simulink model "pedalboys_finalfxchain"  (R2025b)
settings: Solver=VariableStepAuto  StartTime=0.0  StopTime=inf  FixedStep=44100  RelTol=1e-3
libraries: audiodynamicrange x2, audiosources x1, dspsnks4 x1
(part 2 of 2)

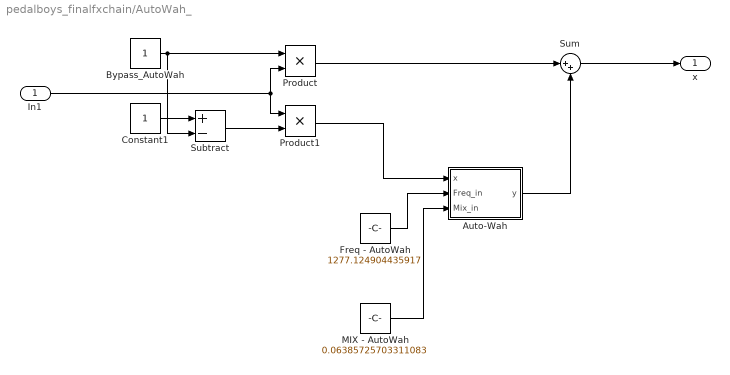
== system pedalboys_finalfxchain/AutoWah_ ==
  In1 : Inport
  Auto-Wah : MATLAB Function  TreatAsAtomicUnit=on
  Bypass_AutoWah : Constant
  Constant1 : Constant
  Freq - AutoWah : Constant  Value=1277.124904435917
  MIX - AutoWah : Constant  Value=0.06385725703311083
  Product : Product
  Product1 : Product
  Subtract : Sum  Inputs=+-
  Sum : Sum  Inputs=|++
  x : Outport
  wires:
  Subtract/1 -> Product1/2
  Bypass_AutoWah/1 -> Product/1, Subtract/2
  Sum/1 -> x/1
  Auto-Wah/1(y) -> Sum/2
  Product/1 -> Sum/1
  In1/1 -> Product/2, Product1/1
  Constant1/1 -> Subtract/1
  Product1/1 -> Auto-Wah/1(x)
  MIX - AutoWah/1 -> Auto-Wah/3(Mix_in)
  Freq - AutoWah/1 -> Auto-Wah/2(Freq_in)

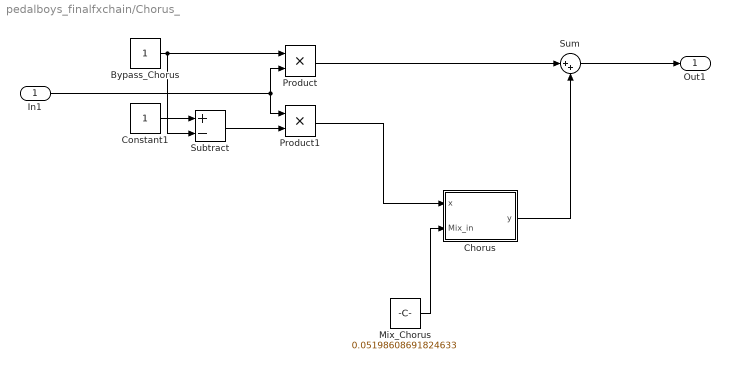
== system pedalboys_finalfxchain/Chorus_ ==
  In1 : Inport
  Bypass_Chorus : Constant
  Chorus : MATLAB Function  TreatAsAtomicUnit=on
  Constant1 : Constant
  Mix_Chorus : Constant  Value=0.05198608691824633
  Product : Product
  Product1 : Product
  Subtract : Sum  Inputs=+-
  Sum : Sum  Inputs=|++
  Out1 : Outport
  wires:
  Product1/1 -> Chorus/1(x)
  Subtract/1 -> Product1/2
  Bypass_Chorus/1 -> Product/1, Subtract/2
  Sum/1 -> Out1/1
  Chorus/1(y) -> Sum/2
  Product/1 -> Sum/1
  In1/1 -> Product/2, Product1/1
  Constant1/1 -> Subtract/1
  Mix_Chorus/1 -> Chorus/2(Mix_in)

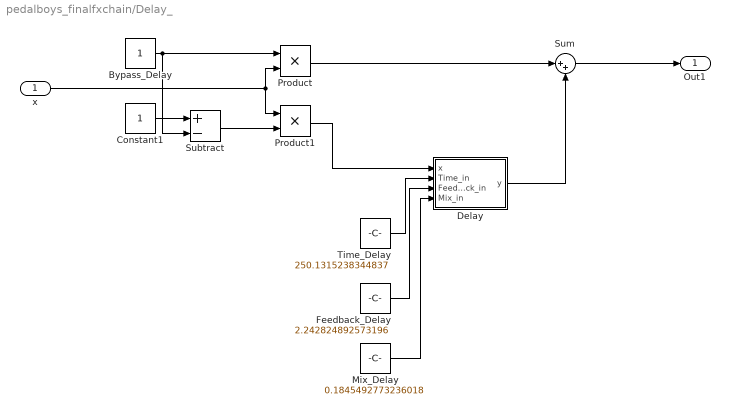
== system pedalboys_finalfxchain/Delay_ ==
  x : Inport
  Bypass_Delay : Constant
  Constant1 : Constant
  Delay : MATLAB Function  TreatAsAtomicUnit=on
  Feedback_Delay : Constant  Value=2.242824892573196
  Mix_Delay : Constant  Value=0.1845492773236018
  Product : Product
  Product1 : Product
  Subtract : Sum  Inputs=+-
  Sum : Sum  Inputs=|++
  Time_Delay : Constant  Value=250.1315238344837
  Out1 : Outport
  wires:
  Sum/1 -> Out1/1
  Product1/1 -> Delay/1(x)
  Product/1 -> Sum/1
  Bypass_Delay/1 -> Product/1, Subtract/2
  Constant1/1 -> Subtract/1
  x/1 -> Product/2, Product1/1
  Subtract/1 -> Product1/2
  Mix_Delay/1 -> Delay/4(Mix_in)
  Time_Delay/1 -> Delay/2(Time_in)
  Feedback_Delay/1 -> Delay/3(Feedback_in)
  Delay/1(y) -> Sum/2

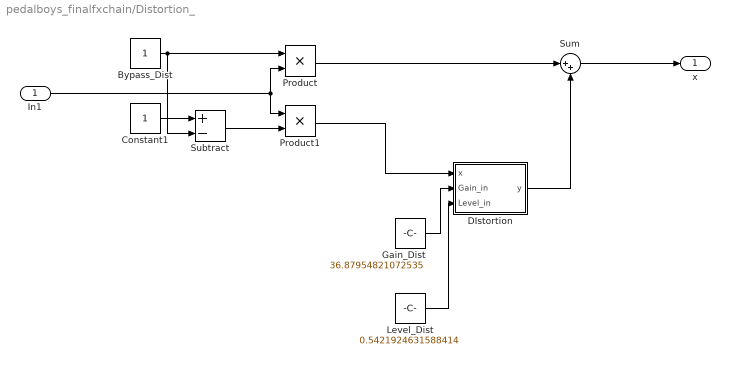
== system pedalboys_finalfxchain/Distortion_ ==
  In1 : Inport
  Bypass_Dist : Constant
  Constant1 : Constant
  DIstortion : MATLAB Function  TreatAsAtomicUnit=on
  Gain_Dist : Constant  Value=36.87954821072535
  Level_Dist : Constant  Value=0.5421924631588414
  Product : Product
  Product1 : Product
  Subtract : Sum  Inputs=+-
  Sum : Sum  Inputs=|++
  x : Outport
  wires:
  Product1/1 -> DIstortion/1(x)
  Subtract/1 -> Product1/2
  Bypass_Dist/1 -> Product/1, Subtract/2
  Sum/1 -> x/1
  DIstortion/1(y) -> Sum/2
  Product/1 -> Sum/1
  In1/1 -> Product/2, Product1/1
  Constant1/1 -> Subtract/1
  Gain_Dist/1 -> DIstortion/2(Gain_in)
  Level_Dist/1 -> DIstortion/3(Level_in)

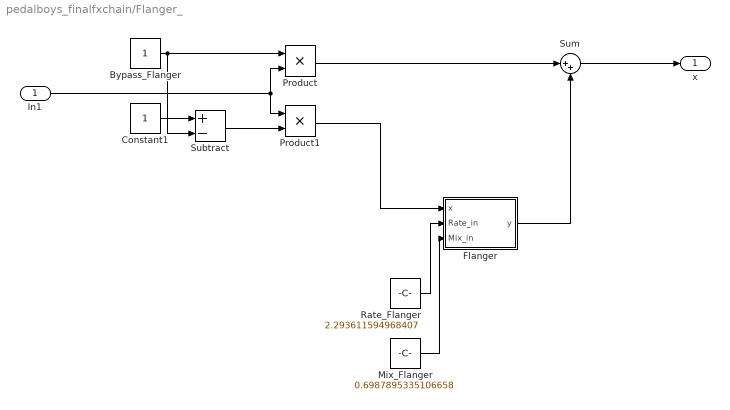
== system pedalboys_finalfxchain/Flanger_ ==
  In1 : Inport
  Bypass_Flanger : Constant
  Constant1 : Constant
  Flanger : MATLAB Function  TreatAsAtomicUnit=on
  Mix_Flanger : Constant  Value=0.6987895335106658
  Product : Product
  Product1 : Product
  Rate_Flanger : Constant  Value=2.293611594968407
  Subtract : Sum  Inputs=+-
  Sum : Sum  Inputs=|++
  x : Outport
  wires:
  Subtract/1 -> Product1/2
  Bypass_Flanger/1 -> Product/1, Subtract/2
  Sum/1 -> x/1
  Flanger/1(y) -> Sum/2
  Product/1 -> Sum/1
  In1/1 -> Product/2, Product1/1
  Constant1/1 -> Subtract/1
  Rate_Flanger/1 -> Flanger/2(Rate_in)
  Product1/1 -> Flanger/1(x)
  Mix_Flanger/1 -> Flanger/3(Mix_in)

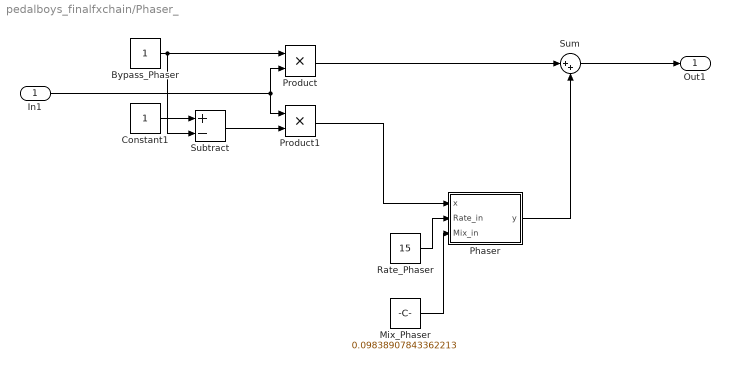
== system pedalboys_finalfxchain/Phaser_ ==
  In1 : Inport
  Bypass_Phaser : Constant
  Constant1 : Constant
  Mix_Phaser : Constant  Value=0.09838907843362213
  Phaser : MATLAB Function  TreatAsAtomicUnit=on
  Product : Product
  Product1 : Product
  Rate_Phaser : Constant  Value=15
  Subtract : Sum  Inputs=+-
  Sum : Sum  Inputs=|++
  Out1 : Outport
  wires:
  Product1/1 -> Phaser/1(x)
  Subtract/1 -> Product1/2
  Bypass_Phaser/1 -> Product/1, Subtract/2
  Sum/1 -> Out1/1
  Phaser/1(y) -> Sum/2
  Product/1 -> Sum/1
  In1/1 -> Product/2, Product1/1
  Constant1/1 -> Subtract/1
  Rate_Phaser/1 -> Phaser/2(Rate_in)
  Mix_Phaser/1 -> Phaser/3(Mix_in)

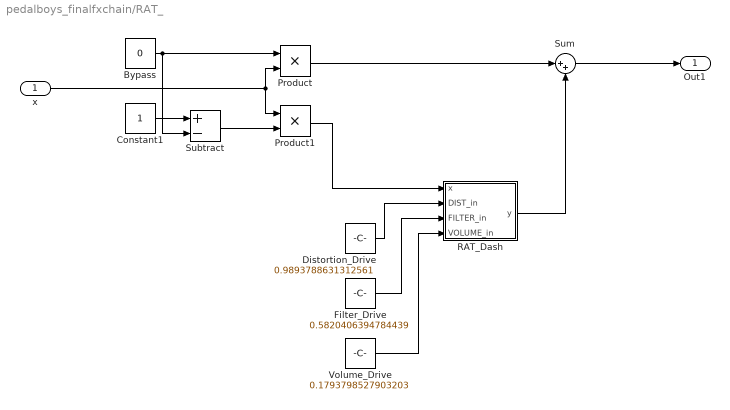
== system pedalboys_finalfxchain/RAT_ ==
  x : Inport
  Bypass : Constant  Value=0
  Constant1 : Constant
  Distortion_Drive : Constant  Value=0.9893788631312561
  Filter_Drive : Constant  Value=0.5820406394784439
  Product : Product
  Product1 : Product
  RAT_Dash : MATLAB Function  TreatAsAtomicUnit=on
  Subtract : Sum  Inputs=+-
  Sum : Sum  Inputs=|++
  Volume_Drive : Constant  Value=0.1793798527903203
  Out1 : Outport
  wires:
  Sum/1 -> Out1/1
  RAT_Dash/1(y) -> Sum/2
  Distortion_Drive/1 -> RAT_Dash/2(DIST_in)
  Volume_Drive/1 -> RAT_Dash/4(VOLUME_in)
  Filter_Drive/1 -> RAT_Dash/3(FILTER_in)
  Product1/1 -> RAT_Dash/1(x)
  Product/1 -> Sum/1
  Bypass/1 -> Product/1, Subtract/2
  Constant1/1 -> Subtract/1
  x/1 -> Product/2, Product1/1
  Subtract/1 -> Product1/2

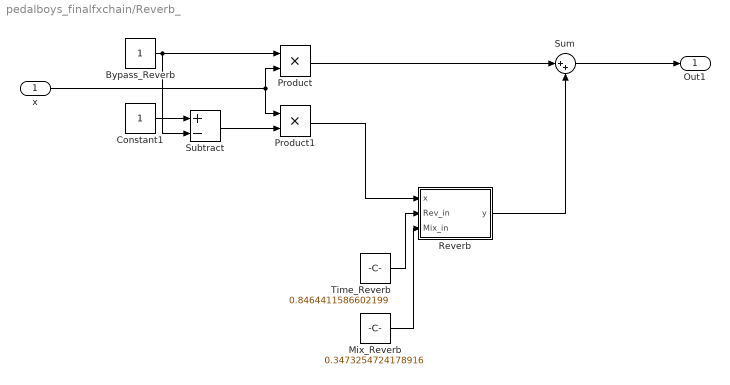
== system pedalboys_finalfxchain/Reverb_ ==
  x : Inport
  Bypass_Reverb : Constant
  Constant1 : Constant
  Mix_Reverb : Constant  Value=0.3473254724178916
  Product : Product
  Product1 : Product
  Reverb : MATLAB Function  TreatAsAtomicUnit=on
  Subtract : Sum  Inputs=+-
  Sum : Sum  Inputs=|++
  Time_Reverb : Constant  Value=0.8464411586602199
  Out1 : Outport
  wires:
  Sum/1 -> Out1/1
  Reverb/1(y) -> Sum/2
  Product1/1 -> Reverb/1(x)
  Product/1 -> Sum/1
  Bypass_Reverb/1 -> Product/1, Subtract/2
  Constant1/1 -> Subtract/1
  x/1 -> Product/2, Product1/1
  Subtract/1 -> Product1/2
  Time_Reverb/1 -> Reverb/2(Rev_in)
  Mix_Reverb/1 -> Reverb/3(Mix_in)

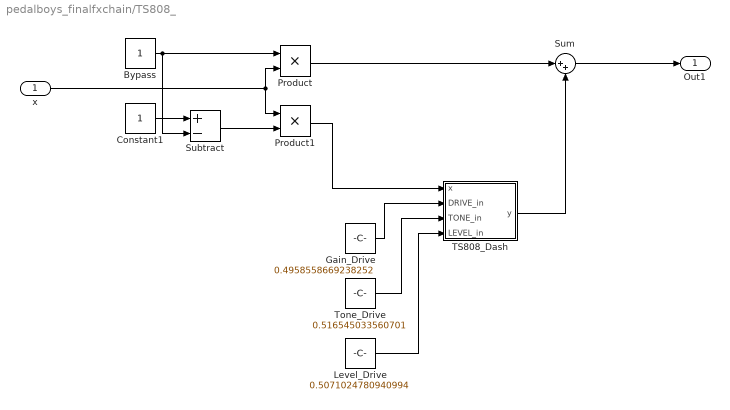
== system pedalboys_finalfxchain/TS808_ ==
  x : Inport
  Bypass : Constant
  Constant1 : Constant
  Gain_Drive : Constant  Value=0.4958558669238252
  Level_Drive : Constant  Value=0.5071024780940994
  Product : Product
  Product1 : Product
  Subtract : Sum  Inputs=+-
  Sum : Sum  Inputs=|++
  TS808_Dash : MATLAB Function  TreatAsAtomicUnit=on
  Tone_Drive : Constant  Value=0.516545033560701
  Out1 : Outport
  wires:
  Sum/1 -> Out1/1
  TS808_Dash/1(y) -> Sum/2
  Gain_Drive/1 -> TS808_Dash/2(DRIVE_in)
  Level_Drive/1 -> TS808_Dash/4(LEVEL_in)
  Tone_Drive/1 -> TS808_Dash/3(TONE_in)
  Product1/1 -> TS808_Dash/1(x)
  Product/1 -> Sum/1
  Bypass/1 -> Product/1, Subtract/2
  Constant1/1 -> Subtract/1
  x/1 -> Product/2, Product1/1
  Subtract/1 -> Product1/2

== matlab function pedalboys_finalfxchain/RAT_/RAT_Dash ==
  data: x input; y output; DIST_in input; FILTER_in input; VOLUME_in input
function y = rat(x, DIST_in, FILTER_in, VOLUME_in)
%#codegen
% ProCo RAT (LM308) 스타일 디스토션 - MATLAB Function 블록용
% 입력:  x (N x 1) mono frame
% 출력:  y (N x 1)

% =========================
% 0) 사용자 파라미터 (노브 3개)  -- 페달과 동일 의미
% =========================
% DIST   : 0.0 ~ 1.0  (R_DIST 0~100kΩ에 매핑)
% FILTER : 0.0 ~ 1.0  (Tone/Filter 컷오프 475 Hz ~ 22.05 kHz(Nyquist Rate))
% VOLUME : 0.0 ~ 1.0  (출력 레벨)
DIST   = DIST_in;   % Distortion (기본값 예시)
FILTER = FILTER_in;   % Filter/Tone (0=밝음, 1=어둡)
VOLUME = VOLUME_in;   % Volume/Level

% =========================
% 상수(회로 근사/샘플레이트)
% =========================
FS         = 44100;         % 모델 샘플레이트와 동일하게
Ts         = 1/FS;

% 입력 HPF (C1=22nF, R2=1M)  fc ≈ 1/(2πR2C1) ≈ 7.2 Hz
HPF_FC     = 7.2;

% LM308 근사: GBW & Slew
GBW_HZ     = 3.0e5;         % LM308 대역폭 근사(300 kHz 근처로 보수적)
SLEW_VuS   = 0.30;          % 0.3 V/µs (Electrosmash 분석 참조)
SLEW_STEP  = SLEW_VuS * 1e6 * Ts;  % 샘플당 허용 변화량 (V 기준)

% 하드클리핑 다이오드 Vf (1N914 실리콘)
Vf         = 0.65;          % ±Vf로 대칭 하드클립

% Filter/Tone LPF 범위 (Electrosmash: ~475 Hz ~ 32 kHz)
TONE_FMIN  = 475;
TONE_FMAX  = FS/2;

% Dist→게인 매핑 (비반전: 1 + Rpot / (R4‖R5))
R4         = 47;            % Ω
R5         = 560;           % Ω
Rpar       = (R4*R5)/(R4+R5);   % ≈ 43.3 Ω
Rpot_max   = 100e3;         % 100 kΩ

% C4 효과(피드백 LPF) 근사: fc ≈ GBW / G  (G↑→fc↓)
% 너무 극단값 방지용 클램프
C4_FC_MIN  = 1200;          % Hz
C4_FC_MAX  = 20000;         % Hz

% 안전 클리핑 한 줄 (디지털 포화)
CLIP_MAX   = 1.0;
CLIP_MIN   = -1.0;

% =========================
% 상태 (persistent)
% =========================
persistent hpf_x1 hpf_y1 ...      % 입력 HPF
           prelp_y1 ...           % C4/GBW 근사용 1차 LPF 출력상태
           slew_prev ...          % Slew limiter 이전 출력
           tone_y1                % Tone 1차 LPF 상태
if isempty(hpf_x1)
    hpf_x1   = 0;  hpf_y1   = 0;
    prelp_y1 = 0;
    slew_prev= 0;
    tone_y1  = 0;
end

% =========================
% 파라미터 매핑
% =========================
% Dist → Rpot (0~100k) → G = 1 + Rpot/Rpar
Rpot  = Rpot_max * max(0,min(1,DIST));        % 0~100k
Gain  = 1 + (Rpot / Rpar);                    % 비반전 이득

% C4/GBW 근사: fc_c4 ≈ GBW / Gain (클램프)
fc_c4 = GBW_HZ / max(Gain,1);
fc_c4 = min(max(fc_c4, C4_FC_MIN), C4_FC_MAX);

% Tone 컷오프 (1차 LPF, 475 Hz ~ 32 kHz)
fc_tone = TONE_FMIN * (TONE_FMAX/TONE_FMIN)^( 1 - max(0,min(1,FILTER)) );
% 0 → TONE_FMAX(밝음), 1 → TONE_FMIN(어둠)

% (지수 매핑: 노브 회전감이 자연스러움)

% 1차 IIR 계수 계산 (bilinear/디지털 1 pole 표준)
alpha_hpf  = exp(-2*pi*HPF_FC*Ts);         % HPF (DC 제거용)
alpha_c4   = exp(-2*pi*fc_c4*Ts);          % C4/GBW 근사 LPF
alpha_tone = exp(-2*pi*fc_tone*Ts);        % Tone LPF

N = size(x,1);
y = zeros(N,1);

for n = 1:N
    xn = x(n);

    % -------------------------
    % 1) 입력 HPF (C1//R2)
    % y = a*y + a*(x - x1)
    y_hpf   = alpha_hpf*hpf_y1 + alpha_hpf*(xn - hpf_x1);
    hpf_x1  = xn;
    hpf_y1  = y_hpf;

    % -------------------------
    % 2) 비반전 증폭 (Gain) + C4/GBW 근사 LPF (1차)
    % 선형 증폭
    pre_amp = Gain * y_hpf;

    % C4/GBW: 1차 저역통과로 하이엔드 soften (출력에 적용)
    pre_lpf = (1-alpha_c4)*pre_amp + alpha_c4*prelp_y1;
    prelp_y1= pre_lpf;

    % -------------------------
    % 3) Slew Rate limiter (LM308: 0.3 V/us)
    % 샘플간 변화량을 ±SLEW_STEP로 제한
    target  = pre_lpf;
    dy      = target - slew_prev;
    if dy >  SLEW_STEP
        y_slew = slew_prev + SLEW_STEP;
    elseif dy < -SLEW_STEP
        y_slew = slew_prev - SLEW_STEP;
    else
        y_slew = target;
    end
    slew_prev = y_slew;

    % -------------------------
    % 4) AC coupling (C7) -- 디지털에서는 이미 DC가 거의 0 → 통과
    %   필요시 초저역 한 번 더 컷:
    %   y_ac = alpha_ac*y_ac_prev + alpha_ac*(y_slew - y_slew_prev)
    y_ac = y_slew;

    % -------------------------
    % 5) 하드클리핑 (D1/D2 to GND)  → ±Vf 대칭 클립
    %    실제 회로는 R6(1k) 뒤 그라운드 클립. 여기서는 레벨만 맞춰 클립.
    if y_ac >  Vf
        y_clip =  Vf;
    elseif y_ac < -Vf
        y_clip = -Vf;
    else
        y_clip = y_ac;
    end

    % -------------------------
    % 6) Tone(Filter) = 1차 LPF (가변 fc)
    tone_out = (1-alpha_tone)*y_clip + alpha_tone*tone_y1;
    tone_y1  = tone_out;

    % -------------------------
    % 7) Volume
    y_lin = VOLUME * tone_out;

    % 안전 포화 (디지털 레일 보호)
    if y_lin > CLIP_MAX
        y(n) = CLIP_MAX;
    elseif y_lin < CLIP_MIN
        y(n) = CLIP_MIN;
    else
        y(n) = y_lin;
    end
end

== matlab function pedalboys_finalfxchain/Phaser_/Phaser ==
  data: x input; y output; Rate_in input; Mix_in input
function y = fx_phaser(x, Rate_in, Mix_in)
%#codegen
% Phaser: cascaded 1st-order all-pass with LFO sweep (freq→a mapping)
% 입력: x (N×1)

% ===== Tunables =====
FS       = 44100;   % 샘플레이트 (모델과 맞추기)
STAGES   = 4;       % all-pass 단계 수
RATE     = Rate_in;     % Hz (LFO 속도)
MIX      = Mix_in;     % 0=dry만, 1=wet만  → phaser는 보통 0.4~0.7
FEEDBACK = 0.4;     % 0~0.7 권장 (깊이 강화)
DEPTH    = 1.0;     % 0~1 (스윕 폭 스케일)
FMIN     = 200;     % Hz  (스윕 하한)
FMAX     = 1800;    % Hz  (스윕 상한)

% ===== States =====
persistent ap_x ap_y phi y_prev a_smooth
if isempty(ap_x)
    ap_x     = zeros(STAGES,1);
    ap_y     = zeros(STAGES,1);
    phi      = 0;
    y_prev   = 0;
    a_smooth = 0;   % 'a' 스무딩(지터 방지)
end

N = size(x,1);
y = zeros(N,1);

for n = 1:N
    % --- LFO: 0..1 사인 → 주파수 범위로 매핑
    phi = phi + 2*pi*RATE/FS; if phi > 2*pi, phi = phi - 2*pi; end
    u   = 0.5*(sin(phi) + 1.0);                    % 0..1
    fc  = FMIN + DEPTH * (FMAX - FMIN) * u;        % Hz sweep
    fc  = min(max(fc, 20), 0.45*FS);               % 안전 범위

    % --- freq → all-pass coeff 'a' (Tustin)
    % 1st-order analog AP: H(s)=(s-wc)/(s+wc); s= (2/T)*(1-z^-1)/(1+z^-1)
    % 결과: H(z)= (a + z^-1)/(1 + a z^-1),  a = (1 - K)/(1 + K),  K = tan(pi*fc/FS)
    K   = tan(pi*fc/FS);
    a   = (1 - K) / (1 + K);
    % 스무딩(속도 너무 빠른 계수 변동 방지)
    a_smooth = 0.15*a + 0.85*a_smooth;
    a        = a_smooth;                            % 최종 계수
    % 안전 클램프
    if a >= 0.999, a = 0.999; elseif a <= -0.999, a = -0.999; end

    % --- 입력 + 피드백
    s = x(n) + FEEDBACK*y_prev;

    % --- all-pass 캐스케이드
    for k = 1:STAGES
        yk     = -a*s + ap_x(k) + a*ap_y(k);   % y[n] = -a x[n] + x[n-1] + a y[n-1]
        ap_x(k)= s;
        ap_y(k)= yk;
        s      = yk;
    end

    wet   = s;
    y(n)  = (1 - MIX)*x(n) + MIX*wet;          % dry/wet 믹스 (필수)
    y_prev= y(n);
end

== matlab function pedalboys_finalfxchain/Distortion_/DIstortion ==
  data: x input; y output; Gain_in input; Level_in input
function y = fx_dist(x, Gain_in, Level_in)
%#codegen
% x: frame (Nx1)
% drive: 입력 게인 1~20
% makeup: 후단 보정 게인 0.5~2
% mix: 0=off, 1=on

gain = Gain_in;
Level = Level_in;
mix = 1;

N = size(x,1);
y = zeros(N,1);
for n = 1:N
    s = gain * x(n);
    sw = tanh(s);               % 소프트 클리핑
    y(n) = (1 - mix)*x(n) + mix*(Level*sw);
end

% 게인 많이 올리면(20정도) 퍼즈소리남!

== matlab function pedalboys_finalfxchain/Flanger_/Flanger ==
  data: x input; y output; Rate_in input; Mix_in input
function y = fx_flanger(x ,Rate_in, Mix_in)
%#codegen
% Short LFO-modulated delay with feedback (원본 flanger 컨셉)

% ===== Tunables =====
FS          = 44100;
MAX_MS      = 2.0;     % 최대 지연(ms) ~ comb spacing
MIN_MS      = 0.2;     % 최소 지연(ms)
RATE        = Rate_in;    % Hz (LFO)
DEPTH       = 1.0;     % 0~1 (지연 변조 폭)
FEEDBACK    = 0.7;     % 0~0.7 권장
WET         = Mix_in;
DRY         = 1-Mix_in;

% ===== Buffer =====
persistent buf p Mmax Mmin phi
if isempty(buf)
    Mmax = max(1, round(FS*MAX_MS/1000));
    Mmin = max(1, round(FS*MIN_MS/1000));
    buf  = zeros(Mmax,1);
    p    = 1;   % write ptr
    phi  = 0;   % LFO phase
end

N = size(x,1);
y = zeros(N,1);

for n = 1:N
    phi = phi + 2*pi*RATE/FS; if phi>2*pi, phi = phi-2*pi; end
    %  delay in [Mmin, Mmax]
    dS  = Mmin + round( ((sin(phi)+1)/2) * DEPTH * (Mmax - Mmin) );
    r   = p - dS; if r < 1, r = r + Mmax; end
    delayed = buf(r);

    % output
    y(n) = DRY*x(n) + WET*(delayed);

    % write with feedback
    buf(p) = x(n) + FEEDBACK*y(n);
    p = p + 1; if p > Mmax, p = 1; end
end

== matlab function pedalboys_finalfxchain/AutoWah_/Auto-Wah ==
  data: x input; y output; Freq_in input; Mix_in input
function y = fx_autowah(x, Freq_in, Mix_in)
%#codegen
% 2nd-order Band-Pass (Backward Euler), f0(t) LFO 모듈레이션

% ===== Tunables =====
FS        = 44100;
F_CENTER  = Freq_in;  % Hz
F_RANGE   = 800;   % Hz sweep depth
WAH_FREQ  = 2;     % Hz (LFO)
Q         = 2;     % 공진
MIX       = Mix_in;   % 0~1 (순수 wah 출력 사용시 1)

Q = max(Q,0.1);

% ===== States =====
persistent y1 y2 x1 x2 phi
if isempty(y1)
    y1 = 0; y2 = 0; x1 = 0; x2 = 0; phi = 0;
end

N = size(x,1);
y  = zeros(N,1);
dT = 1/FS;

for n = 1:N
    phi = phi + 2*pi*WAH_FREQ/FS; if phi>2*pi, phi = phi-2*pi; end
    f0  = F_CENTER + F_RANGE * sin(phi);
    f0  = max(f0, 20);                    % 하한 보호
    w0  = 2*pi*f0;

    A0 = 1 + (w0*dT)/Q + (w0*dT)^2;
    A1 = 2*((w0*dT)^2 - 1)/A0;
    A2 = (1 - (w0*dT)/Q + (w0*dT)^2)/A0;
    B0 = (w0*dT/Q)/A0;  B1 = 0;  B2 = -B0;

    yn = B0*x(n) + B1*x1 + B2*x2 - A1*y1 - A2*y2;
    y(n) = (1 - MIX)*x(n) + MIX*yn;

    x2=x1; x1=x(n); y2=y1; y1=yn;
end

== matlab function pedalboys_finalfxchain/Delay_/Delay ==
  data: x input; y output; Time_in input; Feedback_in input; Mix_in input
function y = fx_delay(x, Time_in, Feedback_in, Mix_in)
%#codegen
% Multi-echo delay: y = x + A0*x[n-D] + FB*y[n-D]
% REPEATS와 TAIL_DB로 피드백 이득을 자동 계산해 반복 횟수 조절
% 입력: x (N×1)

% ===== Tunables =====
FS       = 44100;    % 샘플레이트
D_MS     = Time_in;      % 지연(ms) → 에코 간격
A0       = 0.5;      % 첫 탭(피드포워드) 크기
MIX      = Mix_in;      % 0~1 (dry/wet)
REPEATS  = Feedback_in;        % '들리는' 반복 횟수 목표
TAIL_DB  = -40;      % 마지막 반복의 상대 레벨(dB), 예: -40 dB

% ===== Derived: feedback gain from repeats target =====
% |FB|^REPEATS ≈ 10^(TAIL_DB/20) → FB = 10^(TAIL_DB/(20*REPEATS))
if REPEATS > 0
    FB = 10^(TAIL_DB/(20*REPEATS));
else
    FB = 0;
end
FB = max(min(FB, 0.95), 0);  % 안정성 클램프

% ===== Buffers =====
persistent xbuf ybuf p D
if isempty(xbuf)
    D    = max(1, round(FS*D_MS/1000));
    xbuf = zeros(D,1);   % 입력 x의 지연선
    ybuf = zeros(D,1);   % 출력 y의 지연선(피드백용)
    p    = 1;            % write 포인터
end

N = size(x,1);
y = zeros(N,1);

for n = 1:N
    r   = p;            % D 샘플 전 위치
    xd  = xbuf(r);      % x[n-D]
    yd  = ybuf(r);      % y[n-D]

    wet = x(n) + A0*xd + FB*yd;         % 핵심: 피드포워드 + 피드백
    y(n)= (1 - MIX)*x(n) + MIX*wet;     % 드라이/웻 믹스

    % write & advance
    xbuf(p) = x(n);
    ybuf(p) = y(n);
    p = p + 1; if p > D, p = 1; end
end

== matlab function pedalboys_finalfxchain/Reverb_/Reverb ==
  data: x input; y output; Rev_in input; Mix_in input
function y = fx_reverb(x, Rev_in, Mix_in)
%#codegen
% Schroeder/Moorer 스타일: 병렬 피드백 콤 4개 + 직렬 올패스 2개 + 프리딜레이
% 입력: x (N×1)
% ===== Tunables =====
FS       = 44100;   % 샘플레이트 (모델과 맞추기)
MIX      = Mix_in;    % 0=dry only, 1=wet only
PRED_MS  = 20;      % 프리딜레이(ms): 0~40 추천
RT60     = Rev_in;     % 초(s): 잔향 길이(세기) ← 크게 하면 리버브 강해짐
DAMP     = 0.25;    % 0~0.9: 피드백 내 저역통과 가중치(값↑=어두운 리버브)
APG      = 0.7;     % 올패스 계수(0.5~0.75)

% 콤 지연 (ms) — 약간 서로 소수 차이로
COMB_MS  = [29.7, 37.1, 41.1, 43.7];     % 4개
% 올패스 지연 (ms)
AP_MS    = [5.0, 1.7];

% ===== Derived, init =====
persistent preBuf preP preL ...
           cBuf cP cL cG cLP ...
           apBuf apP apL
if isempty(preBuf)
    % Pre-delay
    preL   = max(1, round(FS*PRED_MS/1000));
    preBuf = zeros(max(preL,1),1); preP = 1;

    % Combs
    nC   = numel(COMB_MS);
    cBuf = cell(nC,1); cP = zeros(nC,1); cL = zeros(nC,1);
    cG   = zeros(nC,1);                      % feedback gain from RT60
    cLP  = zeros(nC,1);                      % damping 1-pole state
    for i=1:nC
        cL(i)   = max(1, round(FS*COMB_MS(i)/1000));
        cBuf{i} = zeros(cL(i),1);
        cP(i)   = 1;
        % g = 10^(-3 * D / (RT60*FS))  (RT60에서 -60dB)
        cG(i)   = 10^(-3 * cL(i) / (RT60*FS));
        % 안전 클램프
        if cG(i) > 0.97, cG(i) = 0.97; end
    end

    % All-pass (serial)
    nA   = numel(AP_MS);
    apBuf= cell(nA,1); apP = zeros(nA,1); apL = zeros(nA,1);
    for k=1:nA
        apL(k)   = max(1, round(FS*AP_MS(k)/1000));
        apBuf{k} = zeros(apL(k),1);
        apP(k)   = 1;
    end
end

N = size(x,1);
y = zeros(N,1);

for n = 1:N
    xn = x(n);

    % --- Pre-delay ---
    if preL > 0
        pdOut      = preBuf(preP);
        preBuf(preP)= xn;
        preP       = preP + 1; if preP > preL, preP = 1; end
    else
        pdOut = xn;
    end

    % --- Parallel feedback combs ---
    combSum = 0;
    for i=1:numel(cL)
        idx = cP(i);
        out = cBuf{i}(idx);           % y[n - L]
        % Damping in feedback (one-pole LP)
        cLP(i) = (1 - DAMP)*out + DAMP*cLP(i);
        % Write: input + g * damped_out
        cBuf{i}(idx) = pdOut + cG(i)*cLP(i);
        % Advance
        idx = idx + 1; if idx > cL(i), idx = 1; end
        cP(i) = idx;
        % Sum parallel outs
        combSum = combSum + out;
    end
    wet = combSum / numel(cL);        % 정규화

    % --- Serial all-pass diffusers (APG, delay apL) ---
    for k=1:numel(apL)
        idx    = apP(k);
        bufOut = apBuf{k}(idx);            % z^-M
        v      = wet + APG*bufOut;
        wet    = bufOut - APG*v;           % all-pass 출력
        apBuf{k}(idx) = v;                 % 내부상태 갱신
        idx    = idx + 1; if idx > apL(k), idx = 1; end
        apP(k) = idx;
    end

    % --- Dry/Wet mix ---
    y(n) = (1 - MIX)*xn + MIX*wet;
end

== matlab function pedalboys_finalfxchain/Chorus_/Chorus ==
  data: x input; y output; Mix_in input
function y = fx_chorus(x, Mix_in)
%#codegen
% Dual-voice chorus with fractional delay (linear interpolation)
% 입력: x (N×1, mono frame)

% ===== Tunables =====
FS      = 44100;   % 샘플레이트 (모델과 맞추기)
MIN_MS  = 8;       % 최소 지연 (ms)  [코러스용: 보통 5~20ms]
MAX_MS  = 20;      % 최대 지연 (ms)
RATE1   = 0.35;    % LFO1 (Hz)
RATE2   = 0.65;    % LFO2 (Hz)
DEPTH   = 1.0;     % 0~1 (모듈레이션 폭 스케일)
WET     = Mix_in;     % wet 비중
DRY     = 1-Mix_in;     % dry 비중 (필요에 따라 0.4~0.7로)

% ===== State =====
persistent buf p Mmin Mmax phi1 phi2
if isempty(buf)
    Mmax = max(1, round(FS*MAX_MS/1000));
    Mmin = max(1, round(FS*MIN_MS/1000));
    buf  = zeros(Mmax,1);
    p    = 1;
    phi1 = 0;
    phi2 = pi;   % 위상 오프셋으로 서로 다른 모션
end

N = size(x,1);
y = zeros(N,1);

for n = 1:N
    % 버퍼에 현재 샘플 기록 (write-first 방식)
    buf(p) = x(n);

    % LFO 진행
    phi1 = phi1 + 2*pi*RATE1/FS; if phi1 > 2*pi, phi1 = phi1 - 2*pi; end
    phi2 = phi2 + 2*pi*RATE2/FS; if phi2 > 2*pi, phi2 = phi2 - 2*pi; end

    % 지연(분수 샘플) 계산
    d1 = Mmin + ((sin(phi1)+1)/2) * DEPTH * (Mmax - Mmin);   % float
    d2 = Mmin + ((sin(phi2)+1)/2) * DEPTH * (Mmax - Mmin);

    % 분수 지연 선형 보간: sample at (p - d)
    % d = Nint + frac  →  (1-frac)*buf[p-Nint] + frac*buf[p-Nint-1]
    % --- voice 1 ---
    Nint1 = floor(d1); frac1 = d1 - Nint1;
    i0 = p - Nint1; if i0 < 1, i0 = i0 + Mmax; end
    i1 = i0 - 1;    if i1 < 1, i1 = i1 + Mmax; end
    c1 = (1-frac1)*buf(i0) + frac1*buf(i1);

    % --- voice 2 ---
    Nint2 = floor(d2); frac2 = d2 - Nint2;
    j0 = p - Nint2; if j0 < 1, j0 = j0 + Mmax; end
    j1 = j0 - 1;    if j1 < 1, j1 = j1 + Mmax; end
    c2 = (1-frac2)*buf(j0) + frac2*buf(j1);

    % mix
    ch = 0.5*(c1 + c2);
    y(n) = DRY*x(n) + WET*ch;

    % 포인터 증가 (circular)
    p = p + 1; if p > Mmax, p = 1; end
end

== matlab function pedalboys_finalfxchain/TS808 ==
  data: x input; y output
function y = fcn(x)
%#codegen
% Ibanez TS808 최종 버전 - 트레블/밝기 억제 및 고음 댐핑 강화
% 목표: TONE_FMAX와 G_MAX를 낮춰 고음역대 배음과 소리의 밝기를 억제, 출력 HPF를 미세 조정하여 정돈된 톤 확보
% 입력:  x (N x 1) mono frame
% 출력:  y (N x 1)

% =========================
% 0) 사용자 지정 파라미터 (노브 3개)
% =========================
% 게인 75%
DRIVE  = 0.75;   
% 톤 55%
TONE   = 0.55;   
% 레벨 60%
LEVEL  = 0.60;   

% =========================
% 상수(회로 근사/샘플레이트)
% =========================
FS         = 44100;         
Ts         = 1/FS;

% 입력 HPF (저음 퍼즈 제거)
HPF_FC_IN  = 1.0;           

% **🛠️ 튜닝 1: 출력 HPF 미세 조정 (톤 정돈)**
HPF_FC_OUT = 25.0;          % 20.0 -> 25.0 Hz (극저역대 잔여 노이즈 정리)

% Vf 및 G_MAX (배음 밸런스)
Vf         = 0.70;         

% **🛠️ 튜닝 2: G_MAX 미세 조정 (밝기 감소)**
G_MAX      = 185;           % 190 -> 185 (고음역대 배음 생성 추가 억제)
G_MIN      = 2.0;           

% **🛠️ 튜닝 3: TONE FMAX 대폭 감소 (트레블/밝기 제거)**
TONE_FMAX  = 5500;          % 6000 -> 5500 Hz (고음 댐핑 최대화)
TONE_FMIN  = 400;           

CLIP_MAX   = 1.0;
CLIP_MIN   = -1.0;

% =========================
% 상태 (persistent)
% =========================
persistent hpf_in_x1 hpf_in_y1 ... 
           tone_y1 ...             
           hpf_out_x1 hpf_out_y1   
if isempty(hpf_in_x1)
    hpf_in_x1  = 0;  hpf_in_y1  = 0;
    tone_y1    = 0;
    hpf_out_x1 = 0; hpf_out_y1 = 0;
end

% =========================
% 파라미터 매핑
% =========================
G_range = log10(G_MAX / G_MIN);
% 게인 계산: 2.0 ~ 185 범위에서 지수적 증가
Gain = G_MIN * 10^(G_range * max(0,min(1,DRIVE))); 

% Tone fc 계산
fc_tone = TONE_FMIN + (TONE_FMAX - TONE_FMIN) * max(0,min(1,TONE));

% 1차 IIR 계수 계산
alpha_hpf_in  = exp(-2*pi*HPF_FC_IN*Ts);
alpha_hpf_out = exp(-2*pi*HPF_FC_OUT*Ts);
alpha_tone    = exp(-2*pi*fc_tone*Ts);

N = size(x,1);
y = zeros(N,1); 

for n = 1:N % 프레임 내 샘플 단위 순차 처리
    xn = x(n);

    % -------------------------
    % 1) 입력 HPF (C1/R1 근사)
    y_hpf_in = alpha_hpf_in*hpf_in_y1 + alpha_hpf_in*(xn - hpf_in_x1);
    hpf_in_x1  = xn;
    hpf_in_y1  = y_hpf_in;

    % -------------------------
    % 2) Op-Amp 증폭 + 피드백 클리핑
    
    % 미드 부스트 계수 (펀치감 보상)
    y_boosted = y_hpf_in * 1.25; 
    
    % 선형 증폭 (G_MAX=185 적용)
    v_in_g = Gain * y_boosted; 

    % atan 클리핑
    clip_level = Vf;
    y_clip_soft = clip_level * atan(v_in_g / clip_level);
    
    y_amp = y_clip_soft; 

    % -------------------------
    % 3) Tone (Filter) = 가변 컷오프 1차 LPF
    tone_out = (1-alpha_tone)*y_amp + alpha_tone*tone_y1;
    tone_y1  = tone_out;

    % -------------------------
    % 4) 출력 HPF (C6/R11 근사)
    y_hpf_out = alpha_hpf_out*hpf_out_y1 + alpha_hpf_out*(tone_out - hpf_out_x1);
    hpf_out_x1  = tone_out;
    hpf_out_y1  = y_hpf_out;
    
    % -------------------------
    % 5) Volume
    y_lin = LEVEL * y_hpf_out;

    % 안전 포화
    if y_lin > CLIP_MAX
        y(n) = CLIP_MAX;
    elseif y_lin < CLIP_MIN
        y(n) = CLIP_MIN;
    else
        y(n) = y_lin;
    end
end

== matlab function pedalboys_finalfxchain/TS808_/TS808_Dash ==
  data: x input; y output; DRIVE_in input; TONE_in input; LEVEL_in input
function y = fcn(x, DRIVE_in, TONE_in, LEVEL_in)
%#codegen
% Ibanez TS808 최종 버전 - Simulink Dashboard 인터페이스용 수정 버전
% 입력:  x (N x 1) mono frame
%        DRIVE_in, TONE_in, LEVEL_in (스칼라) - Simulink Knob 연결용 입력
% 출력:  y (N x 1)

% =========================
% 0) 사용자 지정 파라미터 (노브 3개) - 외부 입력으로 대체
% =========================
DRIVE  = DRIVE_in;   
TONE   = TONE_in;   
LEVEL  = LEVEL_in;   
% =========================
% 상수(회로 근사/샘플레이트)
% =========================
FS         = 44100;         
Ts         = 1/FS;
% 입력 HPF (저음 퍼즈 제거)
HPF_FC_IN  = 1.0;           
% 🛠️ 튜닝 1: 출력 HPF 미세 조정 (톤 정돈)
HPF_FC_OUT = 25.0;          
% Vf 및 G_MAX (배음 밸런스)
Vf         = 0.70;         
% 🛠️ 튜닝 2: G_MAX 미세 조정 (밝기 감소)
G_MAX      = 185;           
G_MIN      = 2.0;           
% 🛠️ 튜닝 3: TONE FMAX 대폭 감소 (트레블/밝기 제거)
TONE_FMAX  = 5500;          
TONE_FMIN  = 400;           
CLIP_MAX   = 1.0;
CLIP_MIN   = -1.0;
% =========================
% 상태 (persistent)
% =========================
persistent hpf_in_x1 hpf_in_y1 ... 
           tone_y1 ...             
           hpf_out_x1 hpf_out_y1   

% ⚠️ Simulink Coder 사용 시 이 부분은 모델의 초기 상태 설정으로 관리하는 것이 좋습니다.
% if isempty(hpf_in_x1)
%     hpf_in_x1  = 0;  hpf_in_y1  = 0;
%     tone_y1    = 0;
%     hpf_out_x1 = 0; hpf_out_y1 = 0;
% end

% 상태 변수가 초기화되지 않은 경우 (첫 호출 시) 0으로 설정
if isempty(hpf_in_x1)
    hpf_in_x1  = 0.0;  hpf_in_y1  = 0.0;
    tone_y1    = 0.0;
    hpf_out_x1 = 0.0; hpf_out_y1 = 0.0;
end

% =========================
% 파라미터 매핑
% =========================
G_range = log10(G_MAX / G_MIN);
% 게인 계산: 2.0 ~ 185 범위에서 지수적 증가
Gain = G_MIN * 10^(G_range * max(0,min(1,DRIVE))); 
% Tone fc 계산
fc_tone = TONE_FMIN + (TONE_FMAX - TONE_FMIN) * max(0,min(1,TONE));
% 1차 IIR 계수 계산
alpha_hpf_in  = exp(-2*pi*HPF_FC_IN*Ts);
alpha_hpf_out = exp(-2*pi*HPF_FC_OUT*Ts);
alpha_tone    = exp(-2*pi*fc_tone*Ts);
N = size(x,1);
y = zeros(N,1); 
for n = 1:N % 프레임 내 샘플 단위 순차 처리
    xn = x(n);
    % -------------------------
    % 1) 입력 HPF (C1/R1 근사)
    y_hpf_in = alpha_hpf_in*hpf_in_y1 + alpha_hpf_in*(xn - hpf_in_x1);
    hpf_in_x1  = xn;
    hpf_in_y1  = y_hpf_in;
    % -------------------------
    % 2) Op-Amp 증폭 + 피드백 클리핑
    
    % 미드 부스트 계수 (펀치감 보상)
    y_boosted = y_hpf_in * 1.25; 
    
    % 선형 증폭 (G_MAX=185 적용)
    v_in_g = Gain * y_boosted; 
    % atan 클리핑
    clip_level = Vf;
    y_clip_soft = clip_level * atan(v_in_g / clip_level);
    
    y_amp = y_clip_soft; 
    % -------------------------
    % 3) Tone (Filter) = 가변 컷오프 1차 LPF
    tone_out = (1-alpha_tone)*y_amp + alpha_tone*tone_y1;
    tone_y1  = tone_out;
    % -------------------------
    % 4) 출력 HPF (C6/R11 근사)
    y_hpf_out = alpha_hpf_out*hpf_out_y1 + alpha_hpf_out*(tone_out - hpf_out_x1);
    hpf_out_x1  = tone_out;
    hpf_out_y1  = y_hpf_out;
    
    % -------------------------
    % 5) Volume
    y_lin = LEVEL * y_hpf_out;
    % 안전 포화
    if y_lin > CLIP_MAX
        y(n) = CLIP_MAX;
    elseif y_lin < CLIP_MIN
        y(n) = CLIP_MIN;
    else
        y(n) = y_lin;
    end
end

== matlab function pedalboys_finalfxchain/MATLAB Function ==
  data: x input; y output
function y = mono2stereo(x)
%#codegen
% x : Mx1 mono frame
% y : Mx2 stereo frame (L=R=mono)

N = size(x,1);
y = zeros(N,2,'like',x);   % 출력 크기를 명시적으로 Mx2로 생성
y(:,1) = x;
y(:,2) = x;
end
